simulink model "DVB_HPA_AWGN"  (R2021b)
settings: Solver=VariableStepAuto  StartTime=0.0  StopTime=1  RelTol=1e-3
libraries: commutil2 x2, commdigbbndapm x2, dspsrcs4 x2, commfilt2 x2, commrfcorlib x1, commchan3 x1, commrandsrc3 x1, commsink2 x1, commrflib2 x1
settings Model: Creator=Martha Ca$h  LastModifiedBy=Martha Ca$h

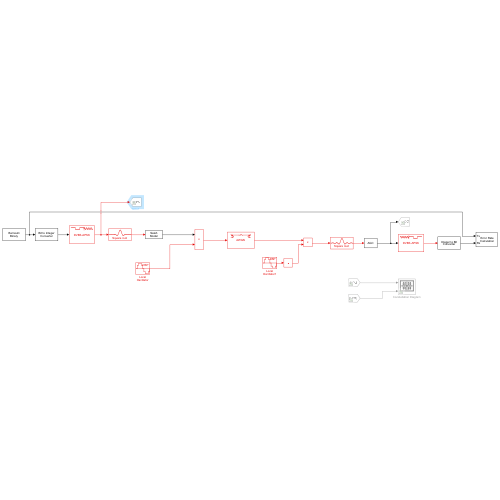
[thumbnail: Simulink's stored preview of the top-level diagram]
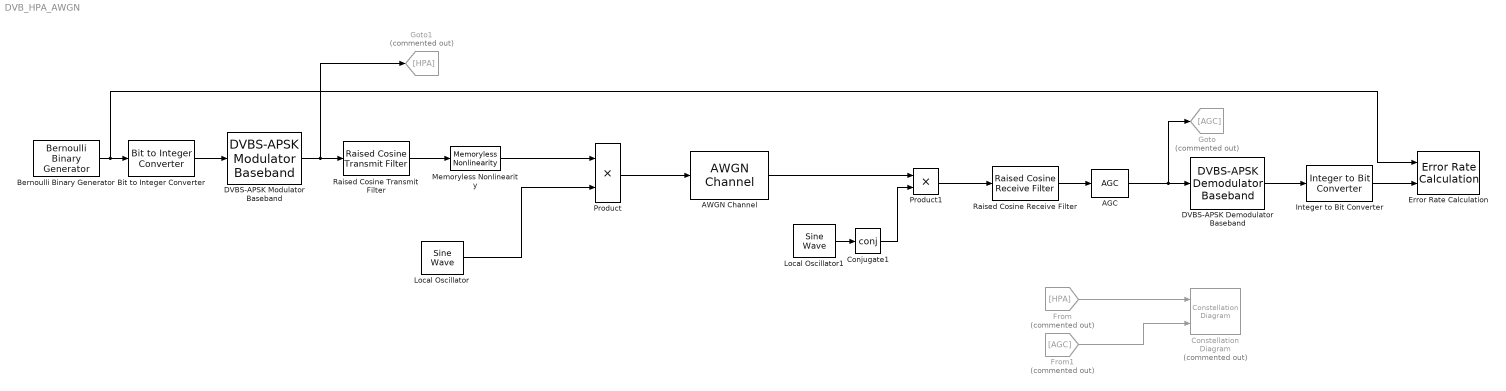
== system DVB_HPA_AWGN ==
  AGC : commrfcorlib/AGC  LegacyMode=off  DetectorMethod=Rectifier  LoopMethod=Linear  UpdatePeriod=100  StepSize=0.1  AdaptationStepSize=0.01  DesiredOutputPower=1  AveragingLength=256  MaximumGain=30  MaxPowerGain=400  GainOutputPort=off  InputPowerOutputPort=off  SimulateUsing=Code generation
  AWGN Channel : commchan3/AWGN Channel  InputProcessing=Columns as channels (frame based)  seed=67  noiseMode="Signal to noise ratio  (Eb/No)"  EbNodB=EbNo  EsNodB=10  SNRdB=10  bitsPerSym=4  Ps=1  Tsym=1e-6  variance=1
  Bernoulli Binary Generator : commrandsrc3/Bernoulli Binary Generator  ProbabilityOfZero=0.5  SeedSource=Auto  Seed=0  SampleTime=1e-6/4  SamplesPerFrame=4  OutputDataType=double  SimulateUsing=Interpreted execution
  Bit to Integer Converter : commutil2/Bit to Integer Converter  nbits=4  bitOrder=MSB first  signedOutputValues=Unsigned  outDtype=Inherit via internal rule  outDtypeSigned=Inherit via internal rule
  Conjugate1 : Math  Operator=conj  SignedPower=on  SaturateOnIntegerOverflow=on
  Constellation Diagram : ConstellationDiagram  Commented=on  NumInputPorts=2
  DVBS-APSK Demodulator Baseband : commdigbbndapm/DVBS-APSK Demodulator Baseband  StdSuffix=S2  FrameLength=Normal  ModOrder=16  CodeIDF=2/3  NormalizationMethod=Outer radius as 1  OutputType=Integer  DecisionType=Hard decision  VarianceSource=Property  NoiseVariance=1  OutputDataType=double  SimulateUsing=Interpreted execution
      settings: SourceProductBaseCode=CM
  DVBS-APSK Modulator Baseband : commdigbbndapm/DVBS-APSK Modulator Baseband  StdSuffix=S2  FrameLength=Normal  ModOrder=16  CodeIDF=2/3  NormalizationMethod=Outer radius as 1  InputType=Integer  OutputDataType=double  SimulateUsing=Code generation
      settings: SourceProductBaseCode=CM
  Error Rate Calculation : commsink2/Error Rate Calculation  N=40  st_delay=0  cp_mode=Entire frame  subframe=[]  PMode=Workspace  WsName=berVec  RsMode2=off  stop=off  numErr=100  maxBits=1e6
  From : From  Commented=on  GotoTag=HPA
  From1 : From  Commented=on  GotoTag=AGC
  Goto : Goto  Commented=on  GotoTag=AGC
  Goto1 : Goto  Commented=on  GotoTag=HPA
  Integer to Bit Converter : commutil2/Integer to Bit Converter  nbits=4  signedInputValues=Unsigned  bitOrder=MSB first  outDtype=Inherit via internal rule
  Local Oscillator : dspsrcs4/Sine Wave  Amplitude=1  Frequency=1.5e9  Phase=0  SampleMode=Discrete  OutComplex=Complex  CompMethod=Trigonometric fcn  TableSize=Speed  SampleTime=(1e-6)/8  SamplesPerFrame=8  ResetState=Restart at time zero  OutputFrames=off  dataType=double  wordLen=16  udDataType=sfix(16)  fracBitsMode=Best precision  numFracBits=15  OutDataTypeStr=double  LastOutDataTypeStr=double
  Local Oscillator1 : dspsrcs4/Sine Wave  Amplitude=1  Frequency=1.5e9  Phase=0  SampleMode=Discrete  OutComplex=Complex  CompMethod=Trigonometric fcn  TableSize=Speed  SampleTime=(1e-6)/8  SamplesPerFrame=8  ResetState=Restart at time zero  OutputFrames=off  dataType=double  wordLen=16  udDataType=sfix(16)  fracBitsMode=Best precision  numFracBits=15  OutDataTypeStr=double  LastOutDataTypeStr=double
  Memoryless Nonlinearity : commrflib2/Memoryless Nonlinearity  model_select=Saleh model  linGaindB=0  GindB=GindB  iip3=30  am2pm=10  LPwrLimAMPM=10  UPwrLimAMPM=inf  amam=[2.1587 1.1517]  ampm=[4.0330 9.1040]  x=[8.1081 1.5413 6.5202 -0.0718]  y=[4.6645 2.0965 10.88 -0.003]  p=0.5  GoutdB=GoutdB  vsat=1
      settings: SourceProductBaseCode=CM
  Product : Product
  Product1 : Product
  Raised Cosine Receive Filter : commfilt2/Raised Cosine Receive Filter  filtType=Square root  R=0.2  filtSpan=10  N=8  downFactor=8  downOffset=0  filterGain=1  InputProcessing=Columns as channels (frame based)  RateOptions=Enforce single-rate processing  framing=Mute  checkCoeff=off  variableName=rcRxFilt  currentFiltSpan=10  D=(10)/2  inputOffset=0  sampMode=Mute  saveAsFlag=0  rateMode=Downsampling  checkGain=Normalized  launchFVT=on  roundingMode=Floor  overflowMode=off  coeffDataTypeStr=Inherit: Same word length as input  coeffMin=[]  coeffMax=[]  coeffLastDataTypeStr=Inherit: Same word length as input  accumDataTypeStr=Inherit: Same as product output  accumLastDataTypeStr=Inherit: Same as product output  outputDataTypeStr=Inherit: Same as accumulator  outputMin=[]  outputMax=[]  outputLastDataTypeStr=Inherit: Same as accumulator
  Raised Cosine Transmit Filter : commfilt2/Raised Cosine Transmit Filter  filtType=Square root  R=0.2  filtSpan=10  N=8  filterGain=1  InputProcessing=Columns as channels (frame based)  RateOptions=Enforce single-rate processing  framing=Mute  checkCoeff=on  variableName=rcTxFilt  checkGain=Normalized  sampMode=Mute  saveAsFlag=0  currentFiltSpan=10  D=(10)/2  launchFVT=on  roundingMode=Floor  overflowMode=off  coeffDataTypeStr=Inherit: Same word length as input  coeffMin=[]  coeffMax=[]  coeffLastDataTypeStr=Inherit: Same word length as input  outputDataTypeStr=Inherit: Same as accumulator  outputMin=[]  outputMax=[]  outputLastDataTypeStr=Inherit: Same as accumulator
  wires:
  AGC/1 -> Goto/1, DVBS-APSK Demodulator Baseband/1
  Conjugate1/1 -> Product1/2
  Bernoulli Binary Generator/1 -> Error Rate Calculation/1, Bit to Integer Converter/1
  Raised Cosine Receive Filter/1 -> AGC/1
  Bit to Integer Converter/1 -> DVBS-APSK Modulator Baseband/1
  Local Oscillator1/1 -> Conjugate1/1
  DVBS-APSK Demodulator Baseband/1 -> Integer to Bit Converter/1
  AWGN Channel/1 -> Product1/1
  Product/1 -> AWGN Channel/1
  Product1/1 -> Raised Cosine Receive Filter/1
  Raised Cosine Transmit Filter/1 -> Memoryless Nonlinearity/1
  DVBS-APSK Modulator Baseband/1 -> Goto1/1, Raised Cosine Transmit Filter/1
  Integer to Bit Converter/1 -> Error Rate Calculation/2
  Local Oscillator/1 -> Product/2
  Memoryless Nonlinearity/1 -> Product/1
  From/1 -> Constellation Diagram/1
  From1/1 -> Constellation Diagram/2
